simulink model "simulacion_algebraico"  (R2020b)
settings: Solver=VariableStepAuto  StartTime=0.0  StopTime=20  RelTol=1e-3
values from neighbouring files (symbols this model uses):
  p0 = x(4)    [ejemplo_6.m]
  p01 = x(6)    [ejemplo_6.m]
  p1 = x(3)    [ejemplo_6.m]
  p11 = x(5)    [ejemplo_6.m]
  p21 = x(4)    [ejemplo_6.m]
  q0 = x(2)    [ejemplo_6.m]
  q01 = x(3)    [ejemplo_6.m]
  q1 = x(1)    [ejemplo_6.m]
  q11 = x(2)    [ejemplo_6.m]
  q21 = x(1)    [ejemplo_6.m]
settings Model: Creator=cmparedes  LastModifiedBy=Acer
settings SFSimCC: CustomCodeUndefinedFunction=UseInterfaceOnly

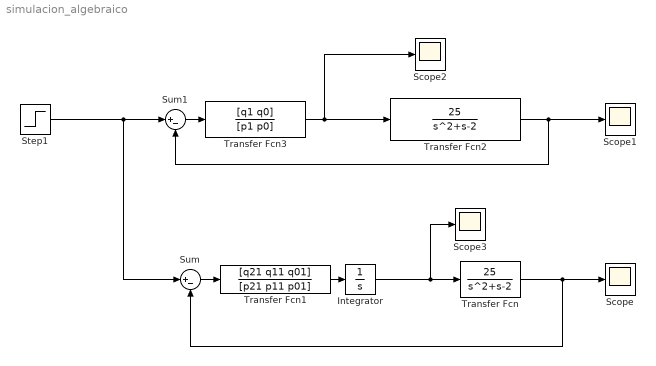
== system simulacion_algebraico ==
  Integrator : Integrator
  Scope{,1..3} (4 alike) : Scope
  Step1 : Step  Time=0  After=10  SampleTime=0
  Sum : Sum  Inputs=|+-
  Sum1 : Sum  Inputs=|+-
  Transfer Fcn : TransferFcn  Numerator=25  Denominator=[1 1 -2]
  Transfer Fcn1 : TransferFcn  Numerator=[q21 q11 q01]  Denominator=[p21 p11 p01]
  Transfer Fcn2 : TransferFcn  Numerator=25  Denominator=[1 1 -2]
  Transfer Fcn3 : TransferFcn  Numerator=[q1 q0]  Denominator=[p1 p0]
  wires:
  Transfer Fcn/1 -> Sum/2, Scope/1
  Sum/1 -> Transfer Fcn1/1
  Transfer Fcn1/1 -> Integrator/1
  Sum1/1 -> Transfer Fcn3/1
  Transfer Fcn2/1 -> Sum1/2, Scope1/1
  Step1/1 -> Sum/1, Sum1/1
  Integrator/1 -> Scope3/1, Transfer Fcn/1
  Transfer Fcn3/1 -> Scope2/1, Transfer Fcn2/1
